simulink library "CTRL_LO_ST4"  (R2023b)
settings: Solver=VariableStepAuto  StartTime=0.0  StopTime=10.0  RelTol=1e-3
undefined symbols (not defined in the file or in its folder): CTRL_LO_p_TqMotLoLim_Nm, CTRL_LO_p_TqMotUpLim_Nm, CTRL_LO_ST4_p_SwtTqFrReRat_na, CTRL_LO_ST4_p_TqFrReRat1_na, CTRL_LO_ST4_p_TqFrReRat2_na, CTRL_LO_ST4_p_TqFrReRat3_na
libraries: simulink x1
settings Model: Creator=blatak  LastModifiedBy=blatak

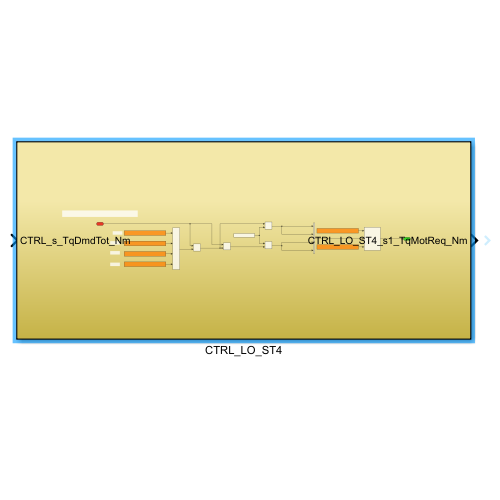
[thumbnail: Simulink's stored preview of the top-level diagram]
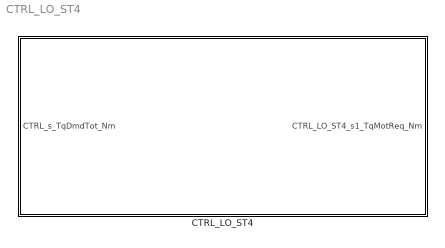
== system CTRL_LO_ST4 ==
  CTRL_LO_ST4 : Subsystem

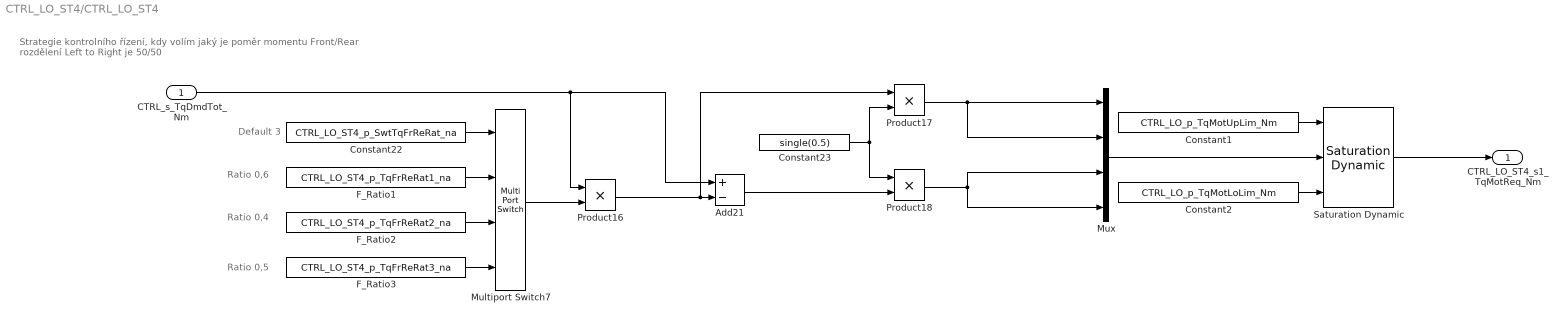
== system CTRL_LO_ST4/CTRL_LO_ST4 ==
  note: Strategie kontrolního řízení, kdy volím jaký je poměr momentu Front/Rear
      | rozdělení Left to Right je 50/50
  note: Ratio 0,6
  note: Default 3
  note: Ratio 0,4
  note: Ratio 0,5
  CTRL_s_TqDmdTot_Nm : Inport
  Add21 : Sum  Inputs=+-
  Constant1 : Constant  Value=CTRL_LO_p_TqMotUpLim_Nm
  Constant2 : Constant  Value=CTRL_LO_p_TqMotLoLim_Nm
  Constant22 : Constant  Value=CTRL_LO_ST4_p_SwtTqFrReRat_na
  Constant23 : Constant  Value=single(0.5)
  F_Ratio1 : Constant  Value=CTRL_LO_ST4_p_TqFrReRat1_na
  F_Ratio2 : Constant  Value=CTRL_LO_ST4_p_TqFrReRat2_na
  F_Ratio3 : Constant  Value=CTRL_LO_ST4_p_TqFrReRat3_na
  Multiport Switch7 : MultiPortSwitch  SaturateOnIntegerOverflow=off  InputSameDT=off
  Mux : Mux
  Product16 : Product
  Product17 : Product
  Product18 : Product
  Saturation Dynamic : simulink/Discontinuities/Saturation Dynamic  OutMin=[]  OutMax=[]  OutDataTypeStr=Inherit: Same as second input  OutDataType=fixdt(1, 16)  OutScaling=2^-10  DoSatur=off
  CTRL_LO_ST4_s1_TqMotReq_Nm : Outport
  wires:
  Product18/1 -> Mux/4, Mux/3
  Constant23/1 -> Product17/2, Product18/1
  Multiport Switch7/1 -> Product16/2
  F_Ratio3/1 -> Multiport Switch7/4
  Product16/1 -> Add21/2, Product17/1
  Product17/1 -> Mux/2, Mux/1
  F_Ratio1/1 -> Multiport Switch7/2
  Add21/1 -> Product18/2
  Constant22/1 -> Multiport Switch7/1
  CTRL_s_TqDmdTot_Nm/1 -> Product16/1, Add21/1
  Saturation Dynamic/1 -> CTRL_LO_ST4_s1_TqMotReq_Nm/1
  F_Ratio2/1 -> Multiport Switch7/3
  Mux/1 -> Saturation Dynamic/2
  Constant1/1 -> Saturation Dynamic/1
  Constant2/1 -> Saturation Dynamic/3
